simulink model "calibTest"  (Simulink 5.0)
settings: Solver=ode1  StartTime=0.0  StopTime=t_stop  FixedStep=T  RelTol=1e-3  AbsTol=1e-6
values from neighbouring files (symbols this model uses):
  calibParams = [469.5 7.95034094731e-05 741.8 8.4355330608e-05 2167.3 0.000136518771331]    [bcc.mat]    (also in calibParams.mat = [471.3 8.26262433661e-05 786 8.69187309865e-05 2173.5 0.0001)
  max1 = 3519.29047619    [20110309T122746.mat]    (also in 20110309T143405.mat; min_max_levels.m = 0.24)
  max2 = 3807.62261905    [20110309T122746.mat]    (also in 20110309T143405.mat; min_max_levels.m = 0.24)
  max3 = 3550.14880952    [20110309T122746.mat]    (also in 20110309T143405.mat; min_max_levels.m = 0.24)
  min1 = 223.146428571    [20110309T122746.mat]    (also in 20110309T143405.mat; min_levels1.m = 0.132; min_max_levels.m = 0.015)
  min2 = 693.047222222    [20110309T122746.mat]    (also in 20110309T143405.mat; min_levels21.m = 0.138; min_levels23.m = 0.135; min_max_levels.m = 0.015)
  min3 = 479.71468254    [20110309T122746.mat]    (also in 20110309T143405.mat; min_levels3.m = 0.135; min_max_levels.m = 0.015)
  T = 0.5    [bcc.mat]    (also in hydrostart.m = 0.25)
  tank1 = [0 0.5 1 1.5 2 2.5 3 3.5 4 4.5 5 5.5 ... (7203 elements, 2401x3)]    [bcc.mat]
  tank2 = [0 0.5 1 1.5 2 2.5 3 3.5 4 4.5 5 5.5 ... (7203 elements, 2401x3)]    [bcc.mat]
  tank3 = [0 0.5 1 1.5 2 2.5 3 3.5 4 4.5 5 5.5 ... (7203 elements, 2401x3)]    [bcc.mat]
undefined symbols (not defined in the file or in its folder): napust, pumps, valves, vypust
libraries: hydro2pumps_lib x1
settings Model: Creator=dmedonza  LastModifiedBy=student  LimitDataPoints=off  BooleanDataType=off  RTWTemplateMakefile=grt_vc.tmf  RTWOptions="-aEnforceIntegerDowncast=1 -aExtMode=0 -aExtModeTesting=0 -aFoldNonRolledExpr=1 -aForceParamTrailComments=0 -aGenerateComments=1 -aGenerateReport=0 -aIgnoreCustomStorageClasses=1 -aIncDataTypeInIds=0 -aIncHierarchyInIds=0 -aInlineInvariantSignals=0 -aInlinedPrmAccess=\"Literals\" -aLocalBlockOutputs=1 -aLogVarNameModifier=\"rt_\" -aMaxRTWIdLen=31 -aPrefixModelToSubsysFcnNames=1 -aRTWVerbose=1 -aRollThreshold=5 -aShowEliminatedStatements=0"

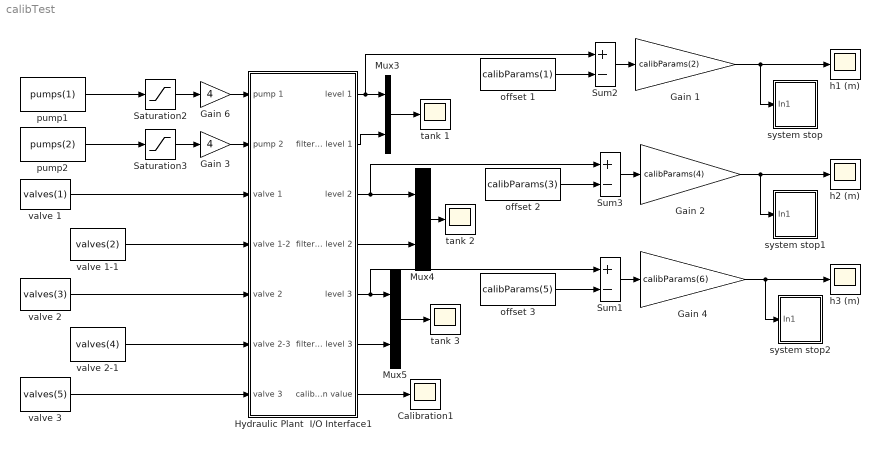
== system calibTest ==
  Calibration1 : Scope
      settings: TickLabels=on  TimeRange=20  YMin=0  YMax=100  SaveName=l  DataFormat=Array
  Gain 1 : Gain  Gain=calibParams(2)  SaturateOnIntegerOverflow=on
  Gain 2 : Gain  Gain=calibParams(4)  SaturateOnIntegerOverflow=on
  Gain 3 : Gain  Gain=4  SaturateOnIntegerOverflow=on
  Gain 4 : Gain  Gain=calibParams(6)  SaturateOnIntegerOverflow=on
  Gain 6 : Gain  Gain=4  SaturateOnIntegerOverflow=on
  Hydraulic Plant  I/O Interface1 : Subsystem
      mask Display: disp('Two Pumps\nHydraulic\nPlant\nI/O Interface')
  Mux3 : Mux  Inputs=2
  Mux4 : Mux  Inputs=2
  Mux5 : Mux  Inputs=2
  Saturation2 : Saturate  UpperLimit=100  LowerLimit=0
  Saturation3 : Saturate  UpperLimit=100  LowerLimit=0
  Sum1 : Sum  Inputs=+-  SaturateOnIntegerOverflow=on
  Sum2 : Sum  Inputs=+-  SaturateOnIntegerOverflow=on
  Sum3 : Sum  Inputs=+-  SaturateOnIntegerOverflow=on
  h1 (m) : Scope
      settings: TickLabels=on  TimeRange=60  YMin=0.238572  YMax=0.263684  SaveName=level1  DataFormat=Array
  h2 (m) : Scope
      settings: TickLabels=on  TimeRange=60  YMin=0.2499  YMax=0.250425  SaveName=level2  DataFormat=Array
  h3 (m) : Scope
      settings: TickLabels=on  TimeRange=60  YMin=0.2561  YMax=0.2571  SaveName=level3  DataFormat=Array
  offset 1 : Constant  Value=calibParams(1)
  offset 2 : Constant  Value=calibParams(3)
  offset 3 : Constant  Value=calibParams(5)
  pump1 : Constant  Value=pumps(1)
  pump2 : Constant  Value=pumps(2)
  system stop : Subsystem
  system stop1 : Subsystem
  system stop2 : Subsystem
  tank 1 : Scope
      settings: TickLabels=on  TimeRange=10  YMin=478  YMax=482  SaveName=tank1  DataFormat=Array  SampleInput=on
  tank 2 : Scope
      settings: TickLabels=on  TimeRange=20  YMin=762.5  YMax=820  SaveName=tank2  DataFormat=Array  SampleInput=on
  tank 3 : Scope
      settings: TickLabels=on  TimeRange=10  YMin=685  YMax=690  SaveName=tank3  DataFormat=Array  SampleInput=on
  valve 1 : Constant  Value=valves(1)
  valve 1-1 : Constant  Value=valves(2)
  valve 2 : Constant  Value=valves(3)
  valve 2-1 : Constant  Value=valves(4)
  valve 3 : Constant  Value=valves(5)
  wires:
  Mux3/1 -> tank 1/1
  Mux5/1 -> tank 3/1
  valve 1/1 -> Hydraulic Plant  I/O Interface1/3(valve 1)
  valve 1-1/1 -> Hydraulic Plant  I/O Interface1/4(valve 1-2)
  valve 2/1 -> Hydraulic Plant  I/O Interface1/5(valve 2)
  valve 2-1/1 -> Hydraulic Plant  I/O Interface1/6(valve 2-3)
  valve 3/1 -> Hydraulic Plant  I/O Interface1/7(valve 3)
  Hydraulic Plant  I/O Interface1/1(level 1) -> Mux3/1, Sum2/1
  Hydraulic Plant  I/O Interface1/2(filtered level 1) -> Mux3/2
  Hydraulic Plant  I/O Interface1/3(level 2) -> Mux4/1, Sum3/1
  Hydraulic Plant  I/O Interface1/4(filtered level 2) -> Mux4/2
  Hydraulic Plant  I/O Interface1/5(level 3) -> Mux5/1, Sum1/1
  Hydraulic Plant  I/O Interface1/6(filtered level 3) -> Mux5/2
  Hydraulic Plant  I/O Interface1/7(calibration value) -> Calibration1/1
  Mux4/1 -> tank 2/1
  offset 1/1 -> Sum2/2
  Sum2/1 -> Gain 1/1
  Gain 6/1 -> Hydraulic Plant  I/O Interface1/1(pump 1)
  Gain 3/1 -> Hydraulic Plant  I/O Interface1/2(pump 2)
  Saturation2/1 -> Gain 6/1
  Saturation3/1 -> Gain 3/1
  offset 2/1 -> Sum3/2
  Sum3/1 -> Gain 2/1
  pump1/1 -> Saturation2/1
  pump2/1 -> Saturation3/1
  Gain 1/1 -> h1 (m)/1, system stop/1(In1)
  Gain 2/1 -> h2 (m)/1, system stop1/1(In1)
  offset 3/1 -> Sum1/2
  Sum1/1 -> Gain 4/1
  Gain 4/1 -> h3 (m)/1, system stop2/1(In1)

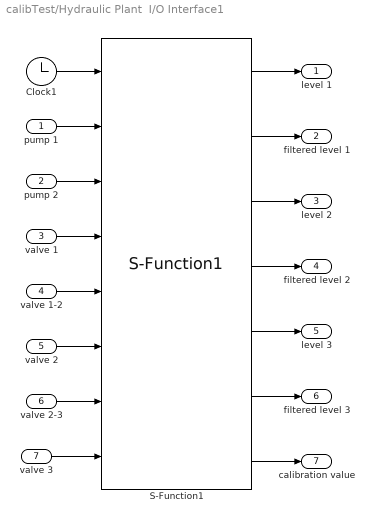
== system calibTest/Hydraulic Plant  I/O Interface1 ==
  pump 1 : Inport
  pump 2 : Inport  Port=2
  valve 1 : Inport  Port=3
  valve 1-2 : Inport  Port=4
  valve 2 : Inport  Port=5
  valve 2-3 : Inport  Port=6
  valve 3 : Inport  Port=7
  Clock1 : Clock
      settings: Decimation=10
  S-Function1 : hydro2pumps_lib/S-Function1  Priority=1  com_port=COM4  Ts=T  events_ot=2  rd_timeout=125  matlab_prior=ABOVE_NORMAL_PRIORITY  warning=on  printout=off
  level 1 : Outport
  filtered level 1 : Outport  Port=2
  level 2 : Outport  Port=3
  filtered level 2 : Outport  Port=4
  level 3 : Outport  Port=5
  filtered level 3 : Outport  Port=6
  calibration value : Outport  Port=7
  wires:
  S-Function1/1 -> level 1/1
  S-Function1/2 -> filtered level 1/1
  Clock1/1 -> S-Function1/1
  pump 1/1 -> S-Function1/2
  pump 2/1 -> S-Function1/3
  S-Function1/3 -> level 2/1
  S-Function1/4 -> filtered level 2/1
  S-Function1/5 -> level 3/1
  S-Function1/6 -> filtered level 3/1
  valve 1/1 -> S-Function1/4
  valve 1-2/1 -> S-Function1/5
  valve 2/1 -> S-Function1/6
  valve 2-3/1 -> S-Function1/7
  S-Function1/7 -> calibration value/1
  valve 3/1 -> S-Function1/8

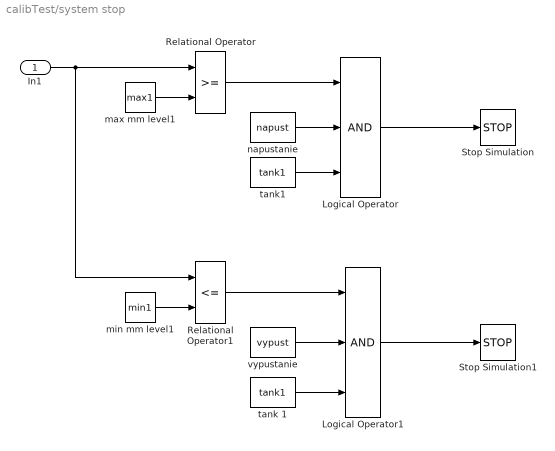
== system calibTest/system stop ==
  In1 : Inport
  Logical Operator : Logic  Inputs=3  AllPortsSameDT=off
  Logical Operator1 : Logic  Inputs=3  AllPortsSameDT=off
  Relational Operator : RelationalOperator
  Relational Operator1 : RelationalOperator  Operator=<=
  Stop Simulation : Stop
  Stop Simulation1 : Stop
  max mm level1 : Constant  Value=max1
  min mm level1 : Constant  Value=min1
  napustanie : Constant  Value=napust
  tank 1 : Constant  Value=tank1
  tank1 : Constant  Value=tank1
  vypustanie : Constant  Value=vypust
  wires:
  In1/1 -> Relational Operator/1, Relational Operator1/1
  max mm level1/1 -> Relational Operator/2
  min mm level1/1 -> Relational Operator1/2
  Relational Operator/1 -> Logical Operator/1
  napustanie/1 -> Logical Operator/2
  Logical Operator/1 -> Stop Simulation/1
  vypustanie/1 -> Logical Operator1/2
  Logical Operator1/1 -> Stop Simulation1/1
  Relational Operator1/1 -> Logical Operator1/1
  tank1/1 -> Logical Operator/3
  tank 1/1 -> Logical Operator1/3

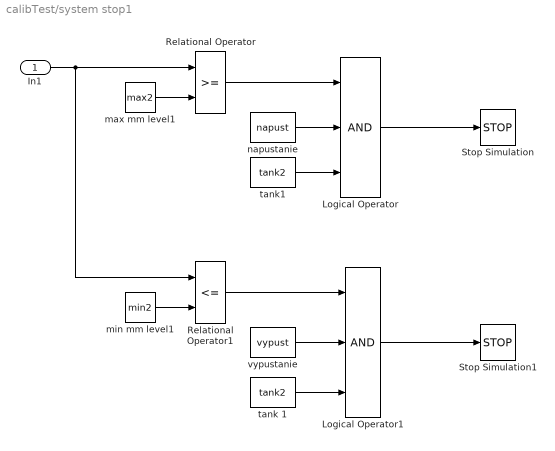
== system calibTest/system stop1 ==
  In1 : Inport
  Logical Operator : Logic  Inputs=3  AllPortsSameDT=off
  Logical Operator1 : Logic  Inputs=3  AllPortsSameDT=off
  Relational Operator : RelationalOperator
  Relational Operator1 : RelationalOperator  Operator=<=
  Stop Simulation : Stop
  Stop Simulation1 : Stop
  max mm level1 : Constant  Value=max2
  min mm level1 : Constant  Value=min2
  napustanie : Constant  Value=napust
  tank 1 : Constant  Value=tank2
  tank1 : Constant  Value=tank2
  vypustanie : Constant  Value=vypust
  wires:
  In1/1 -> Relational Operator/1, Relational Operator1/1
  max mm level1/1 -> Relational Operator/2
  min mm level1/1 -> Relational Operator1/2
  Relational Operator/1 -> Logical Operator/1
  napustanie/1 -> Logical Operator/2
  Logical Operator/1 -> Stop Simulation/1
  vypustanie/1 -> Logical Operator1/2
  Logical Operator1/1 -> Stop Simulation1/1
  Relational Operator1/1 -> Logical Operator1/1
  tank1/1 -> Logical Operator/3
  tank 1/1 -> Logical Operator1/3

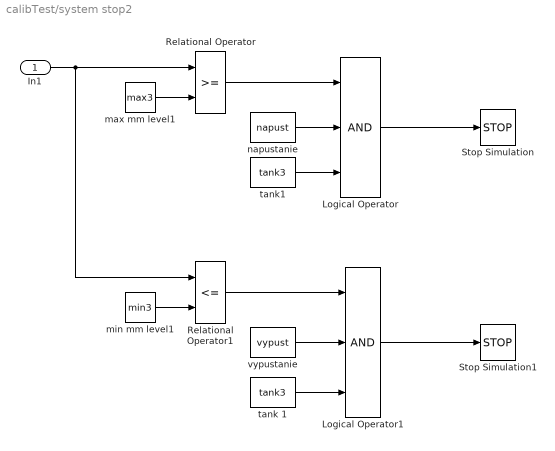
== system calibTest/system stop2 ==
  In1 : Inport
  Logical Operator : Logic  Inputs=3  AllPortsSameDT=off
  Logical Operator1 : Logic  Inputs=3  AllPortsSameDT=off
  Relational Operator : RelationalOperator
  Relational Operator1 : RelationalOperator  Operator=<=
  Stop Simulation : Stop
  Stop Simulation1 : Stop
  max mm level1 : Constant  Value=max3
  min mm level1 : Constant  Value=min3
  napustanie : Constant  Value=napust
  tank 1 : Constant  Value=tank3
  tank1 : Constant  Value=tank3
  vypustanie : Constant  Value=vypust
  wires:
  In1/1 -> Relational Operator/1, Relational Operator1/1
  max mm level1/1 -> Relational Operator/2
  min mm level1/1 -> Relational Operator1/2
  Relational Operator/1 -> Logical Operator/1
  napustanie/1 -> Logical Operator/2
  Logical Operator/1 -> Stop Simulation/1
  vypustanie/1 -> Logical Operator1/2
  Logical Operator1/1 -> Stop Simulation1/1
  Relational Operator1/1 -> Logical Operator1/1
  tank1/1 -> Logical Operator/3
  tank 1/1 -> Logical Operator1/3
